simulink model "control_az7"  (R2019b)
settings: Solver=FixedStepAuto  StartTime=0.0  StopTime=2  FixedStep=1e-5  RelTol=1e-3
settings Model: Creator=SamRayaneh  LastModifiedBy=SamRayaneh
settings DataIOCC: ReturnWorkspaceOutputs=off

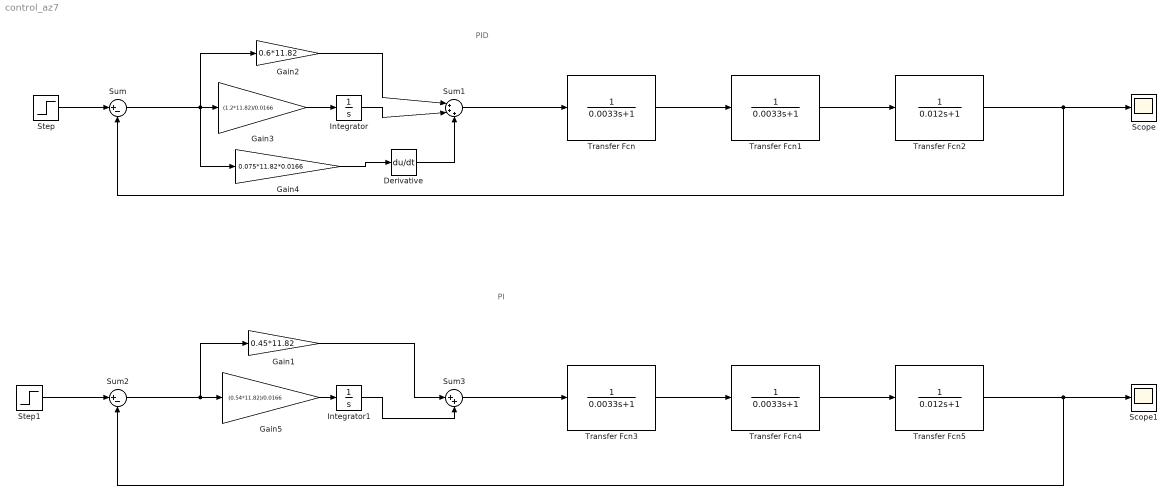
== system control_az7 ==
  note: PI
  note: PID
  Derivative : Derivative
  Gain1 : Gain  Gain=0.45*11.82
  Gain2 : Gain  Gain=0.6*11.82
  Gain3 : Gain  Gain=(1.2*11.82)/0.0166
  Gain4 : Gain  Gain=0.075*11.82*0.0166
  Gain5 : Gain  Gain=(0.54*11.82)/0.0166
  Integrator : Integrator
  Integrator1 : Integrator
  Scope : Scope
  Scope1 : Scope
  Step : Step  Time=0  SampleTime=0
  Step1 : Step  Time=0  SampleTime=0
  Sum : Sum  Inputs=|+-
  Sum1 : Sum  Inputs=|+++
  Sum2 : Sum  Inputs=|+-
  Sum3 : Sum  Inputs=|++
  Transfer Fcn{,1,3..4} (4 alike) : TransferFcn  Denominator=[0.0033 1]
  Transfer Fcn2 : TransferFcn  Denominator=[0.012 1]
  Transfer Fcn5 : TransferFcn  Denominator=[0.012 1]
  wires:
  Transfer Fcn/1 -> Transfer Fcn1/1
  Transfer Fcn1/1 -> Transfer Fcn2/1
  Transfer Fcn2/1 -> Scope/1, Sum/2
  Gain3/1 -> Integrator/1
  Gain4/1 -> Derivative/1
  Sum/1 -> Gain2/1, Gain3/1, Gain4/1
  Gain2/1 -> Sum1/1
  Integrator/1 -> Sum1/2
  Derivative/1 -> Sum1/3
  Sum1/1 -> Transfer Fcn/1
  Sum3/1 -> Transfer Fcn3/1
  Integrator1/1 -> Sum3/2
  Gain1/1 -> Sum3/1
  Sum2/1 -> Gain1/1, Gain5/1
  Gain5/1 -> Integrator1/1
  Transfer Fcn5/1 -> Scope1/1, Sum2/2
  Transfer Fcn4/1 -> Transfer Fcn5/1
  Transfer Fcn3/1 -> Transfer Fcn4/1
  Step1/1 -> Sum2/1
  Step/1 -> Sum/1
